simulink model "CollectionData_Template_2019b"  (R2021a)
settings: Solver=ode1  StartTime=0.0  StopTime=60  FixedStep=0.002  RelTol=1e-3  EnableMultiTasking=on
PostLoadFcn:
  | qc_set_target_type(getConfigSet(bdroot, 'QUARC Default Target Configuration'));
values from neighbouring files (symbols this model uses):
  K_lqr = lqr(sysestc,Q_lqr,R_lqr)    [Compensator_schemes.m]
  v_a_max = 10    [Compensator_schemes.m]
undefined symbols (not defined in the file or in its folder): HIL, k, K_eta, K_x, Kr, L, qc_get_step_size, sysestc
libraries: quarc_library x4, simulink_extras x3, cstblocks x2
settings Model: SimulationMode=external  ExtModeTrigDuration=5000  Creator=CFulford  LastModifiedBy=andre
settings SolverCC: AlgebraicLoopSolver=TrustRegion  PositivePriorityOrder=on
settings DataIOCC: LimitDataPoints=on  SaveFormat=Array  SignalLoggingSaveFormat=ModelDataLogs  ReturnWorkspaceOutputs=off
settings OptimizationCC: ExpressionDepthLimit=2147483647  InitFltsAndDblsToZero=on  LifeSpan=inf
settings DebuggingCC: SaveWithParameterizedLinksMsg=none  UnderspecifiedInitializationDetection=Classic  MergeDetectMultiDrivingBlocksExec=none  SolverPrmCheckMsg=warning  MultiTaskDSMMsg=warning  MultiTaskCondExecSysMsg=none  FcnCallInpInsideContextMsg=warning  StateNameClashWarn=warning  SFUnexpectedBacktrackingDiag=warning  SFNoUnconditionalDefaultTransitionDiag=warning  SFExecutionAtInitializationDiag=none  SFMachineParentedDataDiag=warning  ArithmeticOperatorsInVariantConditions=warning
settings HardwareCC: ProdBitPerPointer=32  ProdBitPerSizeT=32  ProdBitPerPtrDiffT=32  ProdLargestAtomicFloat=None  ProdIntDivRoundTo=Undefined  ProdEndianess=Unspecified  ProdWordSize=32  ProdHWDeviceType=32-bit Generic
settings ModelReferenceCC: PropagateSignalLabelsOutOfModel=off
settings SFSimCC: SimUseLocalCustomCode=off  CustomCodeUndefinedFunction=UseInterfaceOnly
settings RTWCC: Description=QUARC Win64 Target  SystemTargetFile=quarc_win64.tlc  TemplateMakefile=quarc_default_tmf  RTWUseLocalCustomCode=off
settings CodeAppCC: StateflowObjectComments=on
settings STFCustomTargetCC: TargetPreCompLibLocation=C:\PROGRA~3\QUARC\lib\2019b\win64\release  ConcurrentExecutionCompliant=on  CombineOutputUpdateFcns=on  CPPClassGenCompliant=on  GRTInterface=off  UseToolchainInfoCompliant=off  SystemTargetFile=quarc_win64.tlc
settings GRTTargetCC: TargetPreCompLibLocation=C:\PROGRA~3\QUARC\lib\2019b\win64\release  TargetLangStandard=C89/C90 (ANSI)  ParMdlRefBuildCompliant=off  CompOptLevelCompliant=off  MatFileLogging=off  UseToolchainInfoCompliant=off  ExtMode=on  ExtModeMexFile=quarc_comm
settings ConfigComp: CovMetricSettings=dw  CovSaveCumulativeToWorkspaceVar=on  CovSaveSingleToWorkspaceVar=on  CovExternalEMLEnable=off  CovSFcnEnable=off

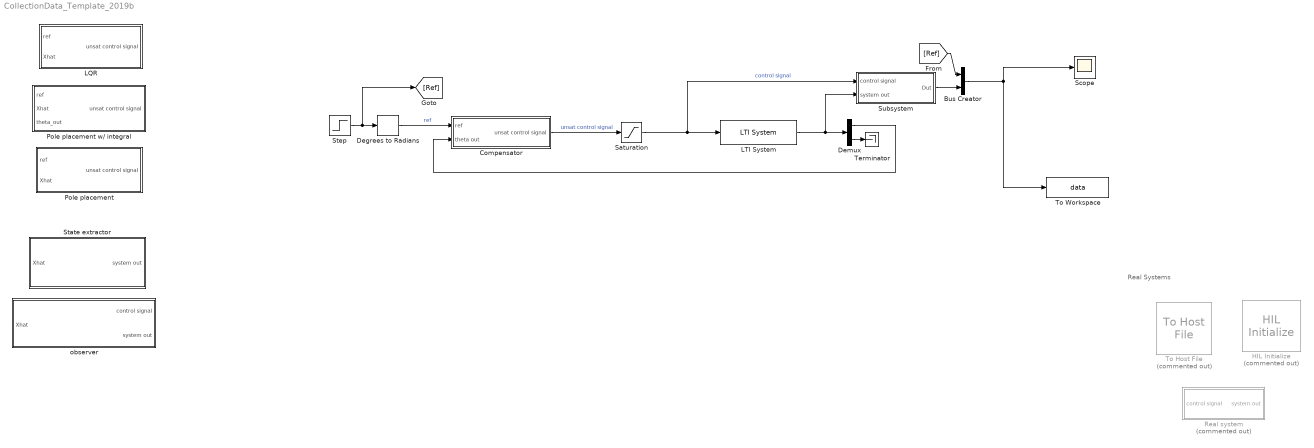
== system CollectionData_Template_2019b ==
  note: Real Systems
  Bus Creator : BusCreator  Inputs=2
  Compensator : Subsystem
  Degrees to Radians : simulink_extras/Transformations/Degrees to Radians
  Demux : Demux  Outputs=2
  HIL Initialize : quarc_library/Data Acquisition/Generic/Configuration/HIL Initialize  Priority=-99  Commented=on  object_name=HIL-1  board_type=q2_usb  board_number=0  board_options=d0=digital;d1=digital;led=auto;update_rate=normal;decimation=1  exclusive=off  active=off  hardware_clocks=[0]  clock_modes=[]  initial_clock_frequencies=[]  set_clock_params_at_start=off  set_clock_params_at_switch_in=off  set_clock_frequencies_at_start=off  set_clock_frequencies_at_switch_in=off  analog_input_channels=[0:1]  analog_input_configurations=[]  analog_input_maximums=10  analog_input_minimums=-10  set_analog_input_params_at_start=on  set_analog_input_params_at_switch_in=off  analog_output_channels=[0:1]  analog_output_maximums=10  analog_output_minimums=-10  initial_analog_outputs=[0]  final_analog_outputs=[0]  watchdog_analog_outputs=0  set_analog_output_params_at_start=on  set_analog_output_params_at_switch_in=off  set_analog_outputs_at_start=on  set_analog_outputs_at_switch_in=off  set_analog_outputs_at_terminate=on  set_analog_outputs_at_switch_out=off  set_analog_outputs_on_watchdog=off  digital_input_channels=[]  digital_output_channels=[]  digital_output_configuration=[]  initial_digital_outputs=[1]  final_digital_outputs=[1]  watchdog_digital_outputs=[1]  set_digital_output_params_at_start=off  set_digital_output_params_at_switch_in=off  set_digital_outputs_at_start=on  set_digital_outputs_at_switch_in=off  set_digital_outputs_at_terminate=on  set_digital_outputs_at_switch_out=off  set_digital_outputs_on_watchdog=off  encoder_channels=[0:1]  quadrature=[4]  encoder_filter_frequency=[]  initial_encoder_counts=[0]  set_encoder_params_at_start=on  set_encoder_params_at_switch_in=off  set_encoder_counts_at_start=on  set_encoder_counts_at_switch_in=off  pwm_channels=[]  pwm_modes=[0]  pwm_frequency=1/0.020  pwm_configuration=[]  pwm_alignment=[]  pwm_polarity=[]  pwm_leading_deadband=[]  pwm_trailing_deadband=[]  initial_pwm_outputs=[0]  final_pwm_outputs=[0]  watchdog_pwm_outputs=[0]  set_pwm_params_at_start=on  set_pwm_params_at_switch_in=off  set_pwm_outputs_at_start=on  set_pwm_outputs_at_switch_in=off  set_pwm_outputs_at_terminate=on  set_pwm_outputs_at_switch_out=off  set_pwm_outputs_on_watchdog=off  other_output_channels=[]  initial_other_outputs=[]  final_other_outputs=[]  watchdog_other_outputs=[]  set_other_outputs_at_start=off  set_other_outputs_at_switch_in=off  set_other_outputs_at_terminate=off  set_other_outputs_at_switch_out=off  set_other_outputs_on_watchdog=off
  LQR : Subsystem
  LTI System : cstblocks/LTI System  sys=sysest  IC=[]
  Pole placement : Subsystem
  Pole placement w/ integral : Subsystem
  Real system : Subsystem  Commented=on
  Saturation : Saturate  UpperLimit=v_a_max  LowerLimit=-v_a_max
  Scope : Scope
  State extractor : Subsystem
  Step : Step  SampleTime=0
  Subsystem : Subsystem
  Terminator : Terminator
  To Host File : quarc_library/Sinks/To Host/To Host File  Commented=on  file_name=Sine tests\Sine_24_in_theta_alpha.mat  variable_name=data  decimation=1  sample_time=-1  file_format=MAT-file v.4  options=No header or footer  append=off  final_file_name=Sine tests\Sine_24_in_theta_alpha.mat  bitrate=2000000
  To Workspace : ToWorkspace  VariableName=data  SampleTime=-1
  observer : Subsystem
  wires:
  Step/1 -> [Ref], Degrees to Radians/1
  Saturation/1 -> LTI System/1, Subsystem/1(control signal)  "control signal"
  Subsystem/1(Out) -> Bus Creator/2
  [Ref] -> Bus Creator/1
  Bus Creator/1 -> To Workspace/1, Scope/1
  LTI System/1 -> Demux/1, Subsystem/2(system out)
  Demux/2 -> Terminator/1
  Demux/1 -> Compensator/2(theta out)
  Degrees to Radians/1 -> Compensator/1(ref)  "ref"
  Compensator/1(unsat control signal) -> Saturation/1  "unsat control signal"

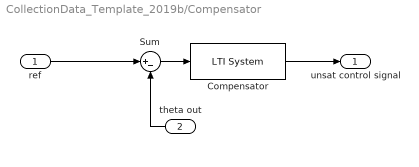
== system CollectionData_Template_2019b/Compensator ==
  ref : Inport
  theta out : Inport  Port=2
  Compensator : cstblocks/LTI System  sys=syscomp_Fire  IC=[]
  Sum : Sum  Inputs=|+-
  unsat control signal : Outport
  wires:
  ref/1 -> Sum/1
  Sum/1 -> Compensator/1
  Compensator/1 -> unsat control signal/1
  theta out/1 -> Sum/2

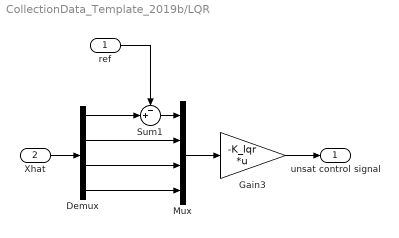
== system CollectionData_Template_2019b/LQR ==
  ref : Inport
  Xhat : Inport  Port=2
  Demux : Demux
  Gain3 : Gain  Gain=-K_lqr  Multiplication=Matrix(K*u)
  Mux : Mux
  Sum1 : Sum  Inputs=-+|
  unsat control signal : Outport
  wires:
  ref/1 -> Sum1/1
  Xhat/1 -> Demux/1
  Demux/1 -> Sum1/2
  Demux/2 -> Mux/2
  Demux/3 -> Mux/3
  Demux/4 -> Mux/4
  Gain3/1 -> unsat control signal/1
  Sum1/1 -> Mux/1
  Mux/1 -> Gain3/1

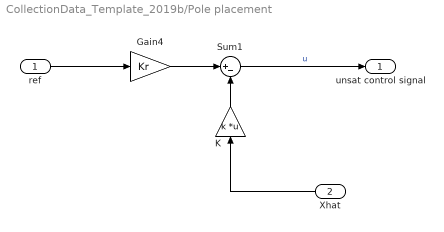
== system CollectionData_Template_2019b/Pole placement ==
  ref : Inport
  Xhat : Inport  Port=2
  Gain4 : Gain  Gain=Kr
  K : Gain  Gain=k  Multiplication=Matrix(K*u)
  Sum1 : Sum  Inputs=|+-
  unsat control signal : Outport
  wires:
  K/1 -> Sum1/2
  Xhat/1 -> K/1
  ref/1 -> Gain4/1
  Sum1/1 -> unsat control signal/1  "u"
  Gain4/1 -> Sum1/1

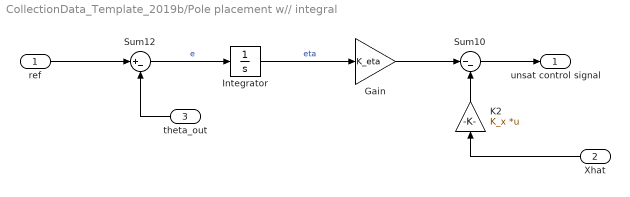
== system CollectionData_Template_2019b/Pole placement w// integral ==
  ref : Inport
  Xhat : Inport  Port=2
  theta_out : Inport  Port=3
  Gain : Gain  Gain=K_eta
  Integrator : Integrator
  K2 : Gain  Gain=K_x  Multiplication=Matrix(K*u)
  Sum10 : Sum  Inputs=|--
  Sum12 : Sum  Inputs=|+-
  unsat control signal : Outport
  wires:
  ref/1 -> Sum12/1
  Gain/1 -> Sum10/1
  Integrator/1 -> Gain/1  "eta"
  Sum10/1 -> unsat control signal/1
  K2/1 -> Sum10/2
  theta_out/1 -> Sum12/2
  Sum12/1 -> Integrator/1  "e"
  Xhat/1 -> K2/1

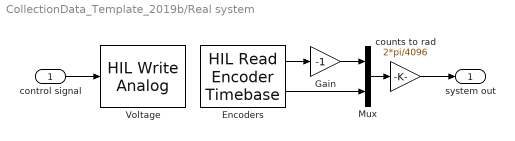
== system CollectionData_Template_2019b/Real system ==
  control signal : Inport
  Encoders : quarc_library/Data Acquisition/Generic/Timebases/HIL Read Encoder Timebase  object_name=HIL-1  clock=0  channels=[0:1]  samples_in_buffer=max(ceil(1/qc_get_step_size), 1)  active=on  vector_output=off  data_type_mode=Inherit via back propagation  data_type=double
  Gain : Gain  Gain=-1
  Mux : Mux  Inputs=2
  Voltage : quarc_library/Data Acquisition/Generic/Immediate I//O/HIL Write Analog  object_name=HIL-1  channels=0  sample_time=-1  active=off  vector_input=off
  counts to rad : Gain  Gain=2*pi/4096
  system out : Outport
  wires:
  control signal/1 -> Voltage/1
  Encoders/1 -> Gain/1
  Encoders/2 -> Mux/2
  Mux/1 -> counts to rad/1
  Gain/1 -> Mux/1
  counts to rad/1 -> system out/1

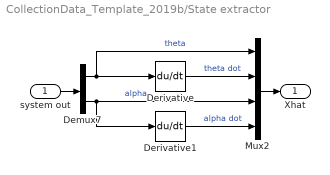
== system CollectionData_Template_2019b/State extractor ==
  system out : Inport
  Demux7 : Demux  Outputs=2
  Derivative : Derivative
  Derivative1 : Derivative
  Mux2 : Mux
  Xhat : Outport
  wires:
  system out/1 -> Demux7/1
  Derivative1/1 -> Mux2/4  "alpha dot"
  Derivative/1 -> Mux2/2  "theta dot"
  Demux7/1 -> Mux2/1, Derivative/1  "theta"
  Demux7/2 -> Derivative1/1, Mux2/3  "alpha"
  Mux2/1 -> Xhat/1

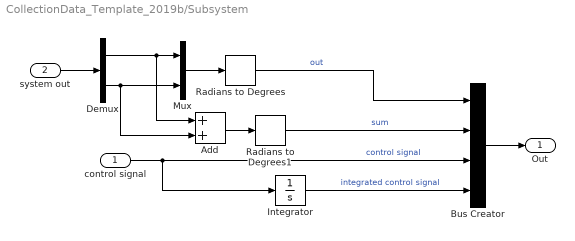
== system CollectionData_Template_2019b/Subsystem ==
  control signal : Inport
  system out : Inport  Port=2
  Add : Sum
  Bus Creator : BusCreator  Inputs=4
  Demux : Demux  Outputs=2
  Integrator : Integrator
  Mux : Mux  Inputs=2
  Radians to Degrees : simulink_extras/Transformations/Radians to Degrees
  Radians to Degrees1 : simulink_extras/Transformations/Radians to Degrees
  Out : Outport
  wires:
  Mux/1 -> Radians to Degrees/1
  control signal/1 -> Integrator/1, Bus Creator/3  "control signal"
  Radians to Degrees1/1 -> Bus Creator/2  "sum"
  Add/1 -> Radians to Degrees1/1
  Radians to Degrees/1 -> Bus Creator/1  "out"
  Integrator/1 -> Bus Creator/4  "integrated control signal"
  Bus Creator/1 -> Out/1
  Demux/2 -> Add/2, Mux/2
  Demux/1 -> Add/1, Mux/1
  system out/1 -> Demux/1

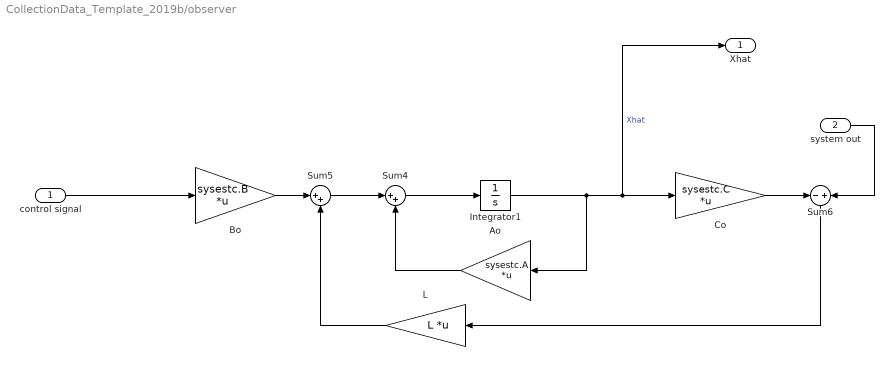
== system CollectionData_Template_2019b/observer ==
  control signal : Inport
  system out : Inport  Port=2
  Ao : Gain  Gain=sysestc.A  Multiplication=Matrix(K*u)
  Bo : Gain  Gain=sysestc.B  Multiplication=Matrix(K*u)
  Co : Gain  Gain=sysestc.C  Multiplication=Matrix(K*u)
  Integrator1 : Integrator
  L : Gain  Gain=L  Multiplication=Matrix(K*u)
  Sum4 : Sum  Inputs=|++
  Sum5 : Sum  Inputs=|++
  Sum6 : Sum  Inputs=-+
  Xhat : Outport
  wires:
  system out/1 -> Sum6/2
  Ao/1 -> Sum4/2
  Sum4/1 -> Integrator1/1
  control signal/1 -> Bo/1
  Co/1 -> Sum6/1
  Sum6/1 -> L/1
  Bo/1 -> Sum5/1
  L/1 -> Sum5/2
  Integrator1/1 -> Xhat/1, Co/1, Ao/1  "Xhat"
  Sum5/1 -> Sum4/1
